simulink model "Nonlinear_parameterchange"  (R2020b)
settings: Solver=ode113  StartTime=0.0  StopTime=1000  RelTol=1e-5
values from neighbouring files (symbols this model uses):
  ap = 1    [Main_Nonlinear.m]
  Gam = 2*diag([1 1 1 1 1 1])    [Main_Nonlinear.m]
  kp = 3    [Main_Nonlinear.m]
  signkp = sign(kp)    [Main_Nonlinear.m]
  theta = [0;0;0;0;0;0]    [Main_Nonlinear.m]
  theta_f = [0.01;-1;1;0.5]    [Main_Nonlinear.m]
libraries: cstblocks x1
settings Model: Creator=Thilo  LastModifiedBy=andrei

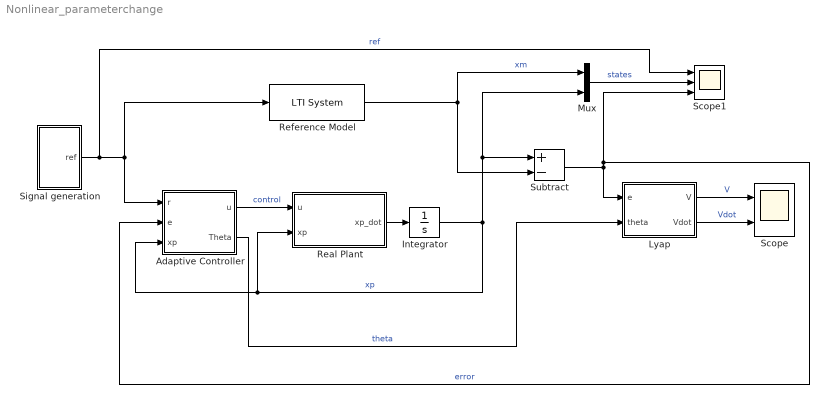
== system Nonlinear_parameterchange ==
  Adaptive Controller : Subsystem
  Integrator : Integrator
  Lyap : MATLAB Function  TreatAsAtomicUnit=on
  Mux : Mux  Inputs=2
  Real Plant : MATLAB Function  TreatAsAtomicUnit=on
  Reference Model : cstblocks/LTI System  sys=M  IC=[0]
  Scope : Scope  NumInputPorts=2
  Scope1 : Scope  NumInputPorts=3
  Signal generation : Subsystem
  Subtract : Sum  Inputs=+-
  wires:
  Integrator/1 -> Subtract/1, Mux/2, Adaptive Controller/3(xp), Real Plant/2(xp)  "xp"
  Adaptive Controller/1(u) -> Real Plant/1(u)  "control"
  Subtract/1 -> Scope1/3, Adaptive Controller/2(e), Lyap/1(e)  "error"
  Reference Model/1 -> Subtract/2, Mux/1  "xm"
  Mux/1 -> Scope1/2  "states"
  Real Plant/1(xp_dot) -> Integrator/1
  Signal generation/1(ref) -> Scope1/1, Adaptive Controller/1(r), Reference Model/1  "ref"
  Adaptive Controller/2(Theta) -> Lyap/2(theta)  "theta"
  Lyap/1(V) -> Scope/1  "V"
  Lyap/2(Vdot) -> Scope/2  "Vdot"

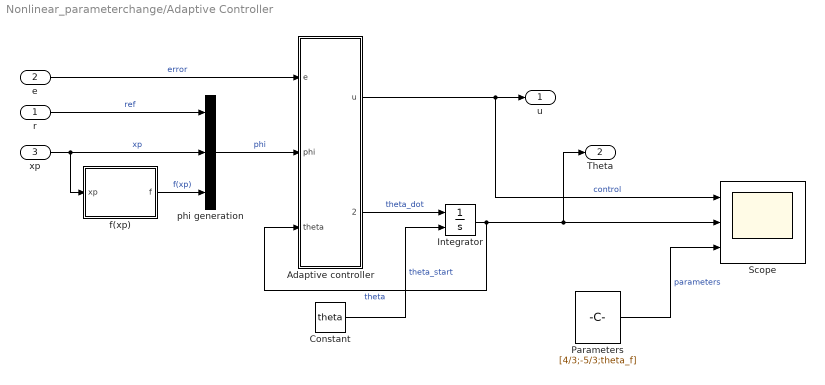
== system Nonlinear_parameterchange/Adaptive Controller ==
  r : Inport
  e : Inport  Port=2
  xp : Inport  Port=3
  Adaptive controller : MATLAB Function  TreatAsAtomicUnit=on
  Constant : Constant  Value=theta
  Integrator : Integrator  InitialConditionSource=external  InitialCondition=[0;0;0]
  Parameters : Constant  Value=[4/3;-5/3;theta_f]
  Scope : Scope  NumInputPorts=3
  "f(xp) " : MATLAB Function  TreatAsAtomicUnit=on
  phi generation : Concatenate  NumInputs=3
  u : Outport
  Theta : Outport  Port=2
  wires:
  r/1 -> phi generation/1  "ref"
  xp/1 -> "f(xp) "/1(xp), phi generation/2  "xp"
  Integrator/1 -> Theta/1, Scope/2, Adaptive controller/3(theta)  "theta"
  e/1 -> Adaptive controller/1(e)  "error"
  Adaptive controller/1(u) -> Scope/1, u/1  "control"
  Constant/1 -> Integrator/2  "theta_start"
  Adaptive controller/2(thetad) -> Integrator/1  "theta_dot"
  Parameters/1 -> Scope/3  "parameters"
  "f(xp) "/1(f) -> phi generation/3  "f(xp)"
  phi generation/1 -> Adaptive controller/2(phi)  "phi"

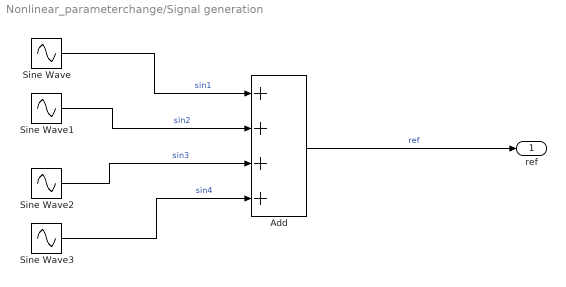
== system Nonlinear_parameterchange/Signal generation ==
  Add : Sum  Inputs=++++
  Sine Wave : Sin  Frequency=3  SampleTime=0
  Sine Wave1 : Sin  Frequency=3/2  SampleTime=0
  Sine Wave2 : Sin  Frequency=3/4  SampleTime=0
  Sine Wave3 : Sin  Frequency=3/8  SampleTime=0
  ref : Outport
  wires:
  Sine Wave/1 -> Add/1  "sin1"
  Sine Wave2/1 -> Add/3  "sin3"
  Sine Wave1/1 -> Add/2  "sin2"
  Sine Wave3/1 -> Add/4  "sin4"
  Add/1 -> ref/1  "ref"

== matlab function Nonlinear_parameterchange/Adaptive Controller/Adaptive controller ==
  data: e input; phi input; u output size=1; theta input size=4; thetad output size=4; signkp parameter; Gam parameter
function [u,thetad] = fcn(e,phi,theta,signkp,Gam)
% Control
u = theta'*phi;
% Adaptive Law
thetad = -Gam* signkp* e* phi;

== matlab function Nonlinear_parameterchange/Adaptive Controller/f(xp)  ==
  data: xp input; f output; theta_f parameter size=2
function f = fcn(xp,theta_f)
% Basis functions
% Second Case
psi_f = [exp(-10*(xp+0.5)^2);exp(-10*(xp-0.5)^2)];
% nonlinear function with unknown gains
f = psi_f;

== matlab function Nonlinear_parameterchange/Real Plant ==
  data: u input; xp_dot output; xp input; kp parameter; ap parameter; theta_f parameter
function xp_dot = fcn(u,xp,kp,ap,theta_f)
% Basis functions of nonlinear function
psi_f = [xp^3;exp(-10*(xp+0.5)^2);exp(-10*(xp-0.5)^2);sin(2*xp)];
% Nonlinear system
if length(theta_f) == 2
    xp_dot = ap*xp+kp*u-kp*[0;theta_f;0]'*psi_f;
else
    xp_dot = ap*xp+kp*u-kp*theta_f'*psi_f;
end

== matlab function Nonlinear_parameterchange/Lyap ==
  data: e input; theta input; V output; Vdot output; Gam parameter; kp parameter; theta_f parameter
function [V, Vdot] = fcn(e,theta,Gam, kp,theta_f)
% Real parameters of plant
theta_star = [4/3;-5/3;theta_f];
% Calculation of parameter error vector
theta_tilde = theta-theta_star;
% Computation of Lyapunv-like function, only possible due to knowledge of real
% parameters
V = 0.5*e^2 + 0.5*abs(kp)*theta_tilde'*inv(Gam)*theta_tilde;
% Negative semi-definite derivative of Lyapunov-like function
Vdot = -4*e^2;
